simulink model "injector_1"  (R2021a)
settings: Solver=VariableStepAuto  StartTime=0.0  StopTime=10.0  RelTol=1e-3
settings Model: Creator=pc  LastModifiedBy=pc

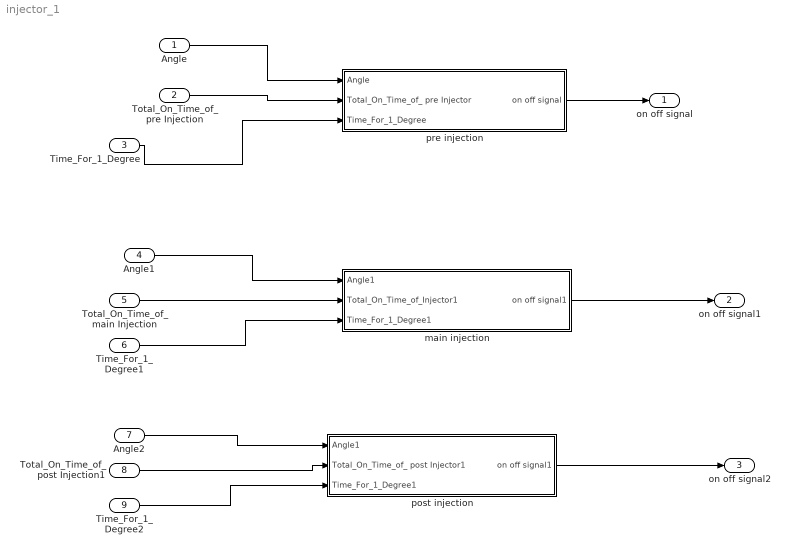
== system injector_1 ==
  Angle : Inport  OutDataTypeStr=single
  Total_On_Time_of_ pre Injection : Inport  Port=2  OutDataTypeStr=single
  Time_For_1_Degree : Inport  Port=3  OutDataTypeStr=single
  Angle1 : Inport  Port=4  OutDataTypeStr=single
  Total_On_Time_of_ main Injection : Inport  Port=5  OutDataTypeStr=single
  Time_For_1_Degree1 : Inport  Port=6  OutDataTypeStr=single
  Angle2 : Inport  Port=7  OutDataTypeStr=single
  Total_On_Time_of_ post Injection1 : Inport  Port=8  OutDataTypeStr=single
  Time_For_1_Degree2 : Inport  Port=9  OutDataTypeStr=single
  main injection : Subsystem
  post injection : Subsystem
  pre injection : Subsystem
  on off signal : Outport  VectorParamsAs1DForOutWhenUnconnected=off
  on off signal1 : Outport  Port=2  VectorParamsAs1DForOutWhenUnconnected=off
  on off signal2 : Outport  Port=3  VectorParamsAs1DForOutWhenUnconnected=off
  wires:
  Angle/1 -> pre injection/1(Angle)
  Total_On_Time_of_ pre Injection/1 -> pre injection/2(Total_On_Time_of_ pre Injector)
  Time_For_1_Degree/1 -> pre injection/3(Time_For_1_Degree)
  pre injection/1(on off signal) -> on off signal/1
  Angle1/1 -> main injection/1(Angle1)
  Total_On_Time_of_ main Injection/1 -> main injection/2(Total_On_Time_of_Injector1)
  Time_For_1_Degree1/1 -> main injection/3(Time_For_1_Degree1)
  main injection/1(on off signal1) -> on off signal1/1
  post injection/1(on off signal1) -> on off signal2/1
  Time_For_1_Degree2/1 -> post injection/3(Time_For_1_Degree1)
  Total_On_Time_of_ post Injection1/1 -> post injection/2(Total_On_Time_of_ post Injector1)
  Angle2/1 -> post injection/1(Angle1)

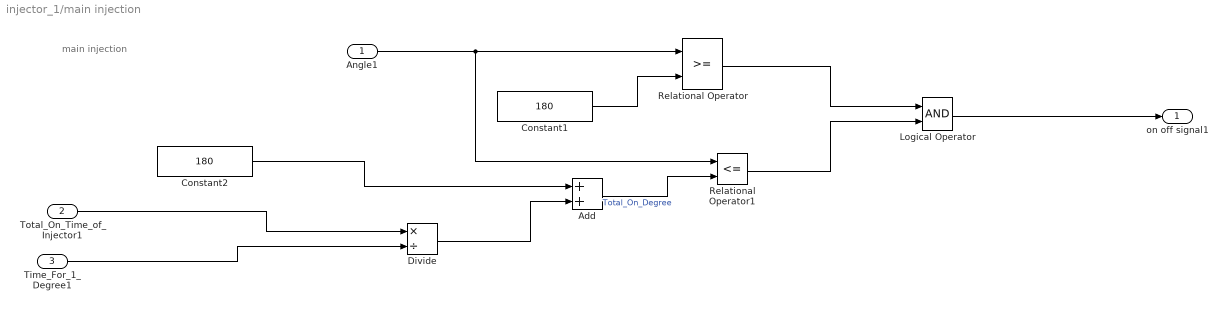
== system injector_1/main injection ==
  note: main injection
  Angle1 : Inport  OutDataTypeStr=single
  Total_On_Time_of_Injector1 : Inport  Port=2  OutDataTypeStr=single
  Time_For_1_Degree1 : Inport  Port=3  OutDataTypeStr=single
  Add : Sum  AccumDataTypeStr=single
      settings: AttributesFormatString=AccumDataTypeStr=%<AccumDataTypeStr>
  Constant1 : Constant  Value=180  OutDataTypeStr=single
  Constant2 : Constant  Value=180  OutDataTypeStr=single
  Divide : Product  Inputs=*/  OutDataTypeStr=single
  Logical Operator : Logic  AllPortsSameDT=off  OutDataTypeStr=boolean
  Relational Operator : RelationalOperator  OutDataTypeStr=boolean  RndMeth=Simplest
  Relational Operator1 : RelationalOperator  Operator=<=  OutDataTypeStr=boolean  RndMeth=Simplest
  on off signal1 : Outport  VectorParamsAs1DForOutWhenUnconnected=off
  wires:
  Logical Operator/1 -> on off signal1/1
  Time_For_1_Degree1/1 -> Divide/2
  Relational Operator/1 -> Logical Operator/1
  Constant2/1 -> Add/1
  Add/1 -> Relational Operator1/2  "Total_On_Degree"
  Angle1/1 -> Relational Operator1/1, Relational Operator/1
  Constant1/1 -> Relational Operator/2
  Relational Operator1/1 -> Logical Operator/2
  Total_On_Time_of_Injector1/1 -> Divide/1
  Divide/1 -> Add/2

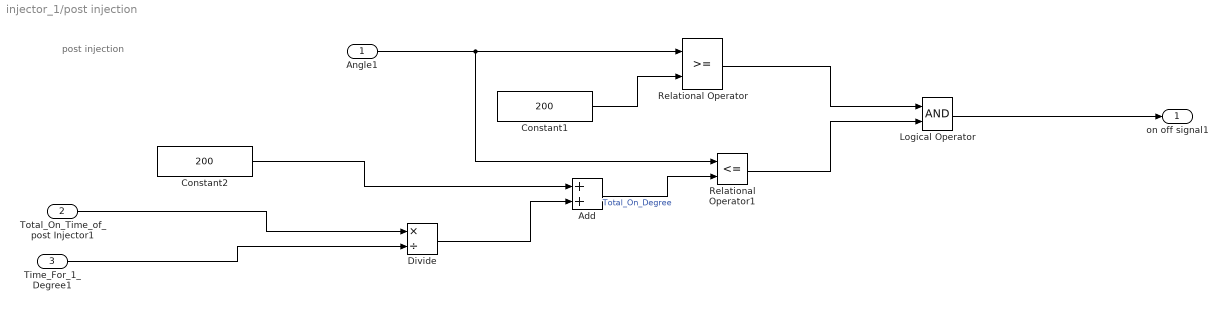
== system injector_1/post injection ==
  note: post injection
  Angle1 : Inport  OutDataTypeStr=single
  Total_On_Time_of_ post Injector1 : Inport  Port=2  OutDataTypeStr=single
  Time_For_1_Degree1 : Inport  Port=3  OutDataTypeStr=single
  Add : Sum  AccumDataTypeStr=single
      settings: AttributesFormatString=AccumDataTypeStr=%<AccumDataTypeStr>
  Constant1 : Constant  Value=200  OutDataTypeStr=single
  Constant2 : Constant  Value=200  OutDataTypeStr=single
  Divide : Product  Inputs=*/  OutDataTypeStr=single
  Logical Operator : Logic  AllPortsSameDT=off  OutDataTypeStr=boolean
  Relational Operator : RelationalOperator  OutDataTypeStr=boolean  RndMeth=Simplest
  Relational Operator1 : RelationalOperator  Operator=<=  OutDataTypeStr=boolean  RndMeth=Simplest
  on off signal1 : Outport  VectorParamsAs1DForOutWhenUnconnected=off
  wires:
  Divide/1 -> Add/2
  Total_On_Time_of_ post Injector1/1 -> Divide/1
  Relational Operator1/1 -> Logical Operator/2
  Constant1/1 -> Relational Operator/2
  Angle1/1 -> Relational Operator/1, Relational Operator1/1
  Add/1 -> Relational Operator1/2  "Total_On_Degree"
  Constant2/1 -> Add/1
  Relational Operator/1 -> Logical Operator/1
  Time_For_1_Degree1/1 -> Divide/2
  Logical Operator/1 -> on off signal1/1

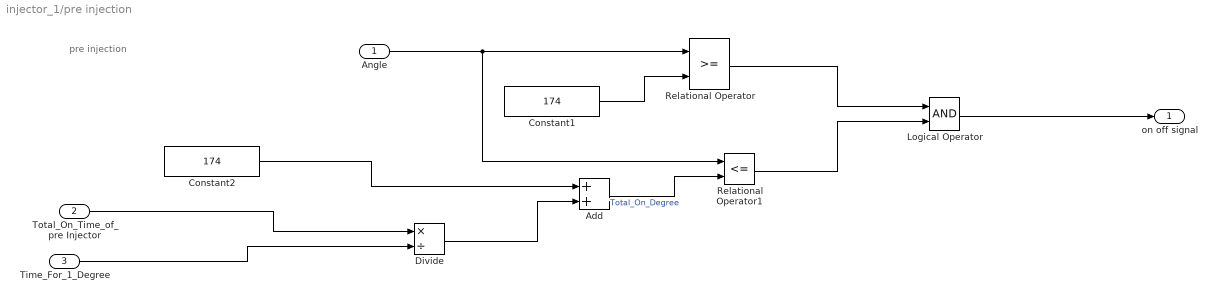
== system injector_1/pre injection ==
  note: pre injection
  Angle : Inport  OutDataTypeStr=single
  Total_On_Time_of_ pre Injector : Inport  Port=2  OutDataTypeStr=single
  Time_For_1_Degree : Inport  Port=3  OutDataTypeStr=single
  Add : Sum  AccumDataTypeStr=single
      settings: AttributesFormatString=AccumDataTypeStr=%<AccumDataTypeStr>
  Constant1 : Constant  Value=174  OutDataTypeStr=single
  Constant2 : Constant  Value=174  OutDataTypeStr=single
  Divide : Product  Inputs=*/  OutDataTypeStr=single
  Logical Operator : Logic  AllPortsSameDT=off  OutDataTypeStr=boolean
  Relational Operator : RelationalOperator  OutDataTypeStr=boolean  RndMeth=Simplest
  Relational Operator1 : RelationalOperator  Operator=<=  OutDataTypeStr=boolean  RndMeth=Simplest
  on off signal : Outport  VectorParamsAs1DForOutWhenUnconnected=off
  wires:
  Divide/1 -> Add/2
  Relational Operator1/1 -> Logical Operator/2
  Constant1/1 -> Relational Operator/2
  Total_On_Time_of_ pre Injector/1 -> Divide/1
  Add/1 -> Relational Operator1/2  "Total_On_Degree"
  Constant2/1 -> Add/1
  Time_For_1_Degree/1 -> Divide/2
  Relational Operator/1 -> Logical Operator/1
  Angle/1 -> Relational Operator1/1, Relational Operator/1
  Logical Operator/1 -> on off signal/1
